simulink model "prvish"  (Simulink 7.8)
settings: Solver=ode45  StartTime=0.0  StopTime=100  RelTol=1e-3
settings Model: Creator=iki  LastModifiedBy=iki

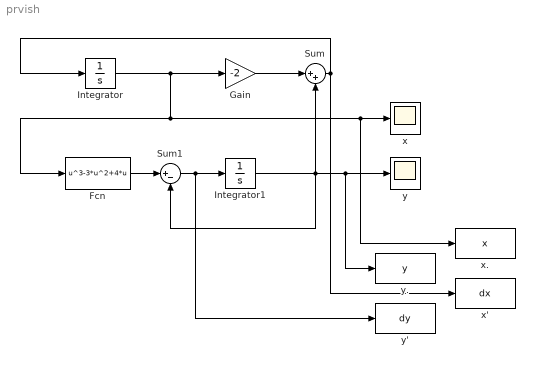
== system prvish ==
  Fcn : Fcn  Expr=u^3-3*u^2+4*u
  Gain : Gain  Gain=-2
  Integrator : Integrator  InitialCondition=0.9
  Integrator1 : Integrator  InitialCondition=3.9
  Sum : Sum  Inputs=|++
  Sum1 : Sum  Inputs=|+-
  x : Scope
  x' : ToWorkspace  VariableName=dx  SampleTime=-1  SaveFormat=Array
  x. : ToWorkspace  VariableName=x  SampleTime=-1  SaveFormat=Array
  y : Scope
  y' : ToWorkspace  VariableName=dy  SampleTime=-1  SaveFormat=Array
  y. : ToWorkspace  VariableName=y  SampleTime=-1  SaveFormat=Array
  wires:
  Integrator/1 -> Gain/1, Fcn/1, x/1, x./1
  Gain/1 -> Sum/1
  Sum/1 -> Integrator/1, x'/1
  Integrator1/1 -> Sum/2, Sum1/2, y/1, y./1
  Sum1/1 -> Integrator1/1, y'/1
  Fcn/1 -> Sum1/1
